simulink model "buckconverter"  (R2022a)
settings: Solver=VariableStepAuto  StartTime=0.0  StopTime=0.7  FixedStep=0.00001  RelTol=1e-3
InitFcn:
  | if ~exist('dx', 'var')
  |     dx = 0.01;
  | else
  |     dx = min(0.01 + 0.05, 1);
  | end
undefined symbols (not defined in the file): dc
libraries: spsSeriesRLCBranchLib x3, spsVoltageMeasurementLib x1, spsDCVoltageSourceLib x1, spsDiodeLib x1, spsCurrentMeasurementLib x1, spsMosfetLib x1, spsMeanLib x1, spsPWMGeneratorDCDCLib x1, spspowerguiLib x1
settings Model: Creator=edgar  LastModifiedBy=edgar
settings DataIOCC: ReturnWorkspaceOutputs=off

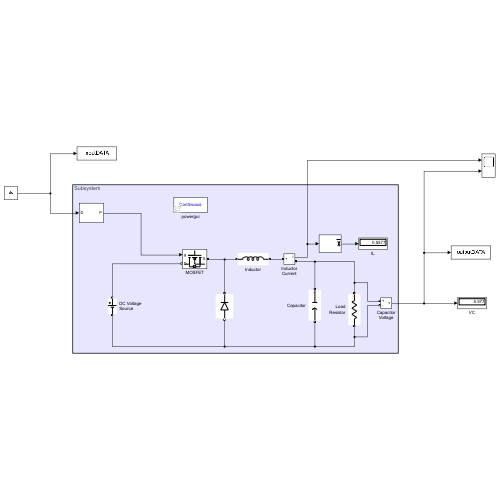
[thumbnail: Simulink's stored preview of the top-level diagram]
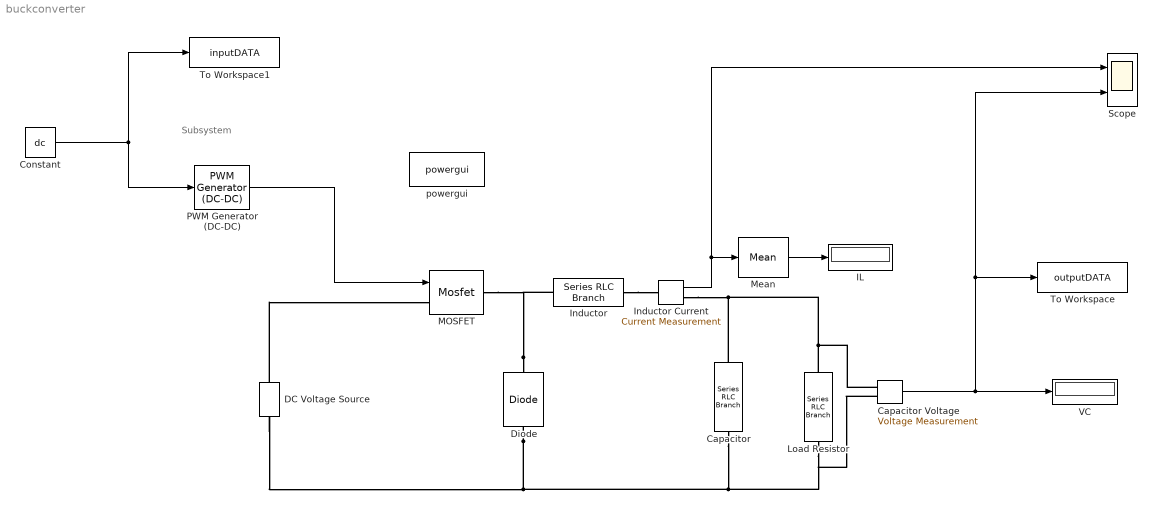
== system buckconverter ==
  note: Subsystem
  Capacitor : spsSeriesRLCBranchLib/Series RLC Branch  LConnTagsString=__new0  RConnTagsString=__new0  BranchType=C  Resistance=1  Inductance=1e-3  SetiL0=off  InitialCurrent=0  Capacitance=220e-6  Setx0=off  InitialVoltage=0  Measurements=None
  Capacitor Voltage : spsVoltageMeasurementLib/Voltage Measurement  PhasorSimulation=off  OutputType=Complex  PSBequivalent=0
  Constant : Constant  Value=dc
  DC Voltage Source : spsDCVoltageSourceLib/DC Voltage Source  Amplitude=12  Measurements=None
  Diode : spsDiodeLib/Diode  Ron=0.001  Lon=0  Vf=0.8  IC=0  UseSnubber=off  Rs=0  Cs=0  Measurements=off
  IL : Display
  Inductor : spsSeriesRLCBranchLib/Series RLC Branch  LConnTagsString=__new0  RConnTagsString=__new0  BranchType=L  Resistance=1  Inductance=0.003  SetiL0=off  InitialCurrent=0  Capacitance=1e-6  Setx0=off  InitialVoltage=0  Measurements=None
  Inductor Current : spsCurrentMeasurementLib/Current Measurement  PhasorSimulation=off  OutputType=Complex  PSBequivalent=0
  Load Resistor : spsSeriesRLCBranchLib/Series RLC Branch  LConnTagsString=__new0  RConnTagsString=__new0  BranchType=R  Resistance=10  Inductance=1e-3  SetiL0=off  InitialCurrent=0  Capacitance=1e-6  Setx0=off  InitialVoltage=0  Measurements=None
  MOSFET : spsMosfetLib/Mosfet  Ron=0.1  Lon=0  Rd=0.01  Vfd=0  IC=0  Rs=1e5  Cs=inf  Measurements=off
  Mean : spsMeanLib/Mean  Freq=5e3  Vinit=0  Ts=0
  PWM Generator (DC-DC) : spsPWMGeneratorDCDCLib/PWM Generator (DC-DC)  Fsw=5000  Ts=0
  Scope : Scope  NumInputPorts=2
  To Workspace : ToWorkspace  VariableName=outputDATA  SampleTime=-1
      settings: Save2DSignal=2-D array (concatenate along first dimension)
  To Workspace1 : ToWorkspace  VariableName=inputDATA  SampleTime=-1
      settings: Save2DSignal=2-D array (concatenate along first dimension)
  VC : Display
  powergui : spspowerguiLib/powergui  Priority=1  SimulationMode=Continuous  SampleTime=50e-6  frequency=60  Iterations=50  frequencyindice=0  Pbase=100e6  ErrMax=1e-4  UnitsV=kV  UnitsW=MW  buscounter=0  FunctionMessages=off  echomessages=off  EnableUseOfTLC=off  CurrentSourceSwitches=on  DisableSnubberDevices=off  DisableRonSwitches=off  DisableVfSwitches=off  DisplayEquations=off  AutomaticDiscreteSolvers=off  SolverType=Tustin  Interpol=off  ExternalGateDelay=off  methode=off  Ts=0  x0status=blocks  SPID=off  SwTol=0  HookPort=off  NonlinearTolerance=1e-4  nMaxIteration=100  ContinueOnMaxIteration=off  RestoreLinks=warning  ResistiveCurrentMeasurement=off  Frange=[0:2:500]  Ylog=off  Xlog=on  ShowGrid=off  save=off  variable=ZData  structure=0  ZoomFFT=off  StartTime=0.0  cycles=1  DisplayStyle=1  fundamental=60  FreqAxis=off  MaxFrequency=1000  frequencyindicesteady=1  RmsSteady=1  display=off
  wires:
  Capacitor Voltage/1 -> Scope/2, To Workspace/1, VC/1
  Inductor Current/1 -> Scope/1, Mean/1
  Constant/1 -> PWM Generator (DC-DC)/1, To Workspace1/1
  Mean/1 -> IL/1
  PWM Generator (DC-DC)/1 -> MOSFET/1
  connections:
  Inductor/RConn1 -- Inductor Current/LConn1
  Diode/LConn1 -- DC Voltage Source/LConn1 -- Capacitor Voltage/LConn2 -- Load Resistor/RConn1 -- Capacitor/RConn1
  Capacitor Voltage/LConn1 -- Load Resistor/LConn1 -- Inductor Current/RConn1 -- Capacitor/LConn1
  Diode/RConn1 -- MOSFET/RConn1 -- Inductor/LConn1
  DC Voltage Source/RConn1 -- MOSFET/LConn1
